simulink model "mainfile"  (R2016a)
settings: Solver=VariableStepAuto  StartTime=0.0  StopTime=3  RelTol=1e-3
undefined symbols (not defined in the file): Acid, Lead
libraries: powerlib x39, powerlib_meascontrol x6, simulink x3, electricdrivelib x1
settings Model: Creator=rinkesh.pee14  LastModifiedBy=rinkesh.pee14

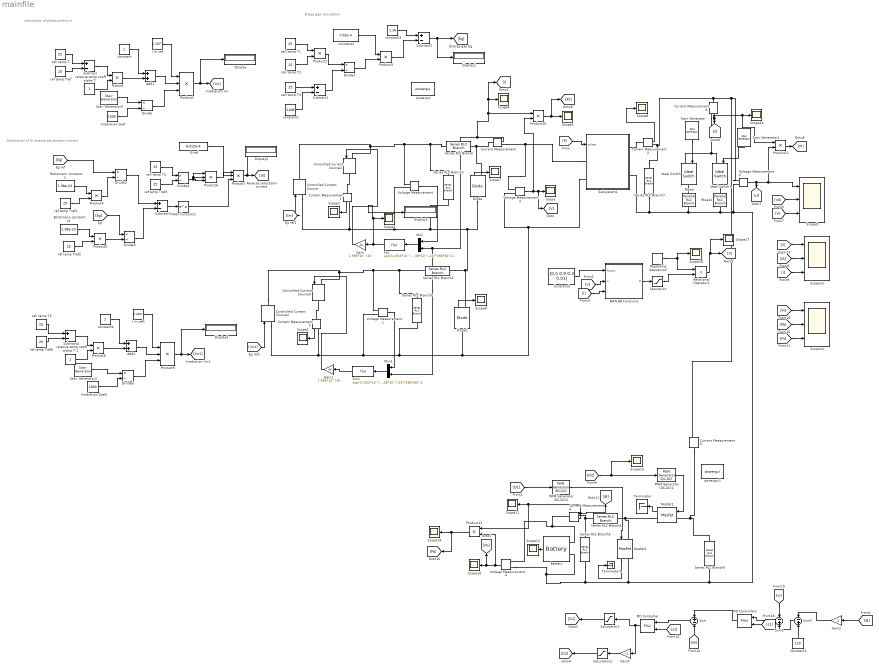
== system mainfile ==
  note: calculation of photocurrent Irr
  note: Enegy gap calculation
  note: Calculation of I0 reverse satuaration current
  Add1 : Sum
  Add2 : Sum
  Battery : electricdrivelib/Extra Sources/Battery  BatType=Lead-Acid  ShowTempParam=off  ThermalPreset=no  NomV=48  NomQ=50  SOC=50  Batt_Tr=30  PresetModel=on  MaxQ=52.0833  MinV=36  FullV=52.2632  Dis_rate=10  R=0.0096  Normal_OP=15.5139  expZone="[48.8684     0.166667]"  current=[1.5 3]  Units=Ampere-hour  Tci=20  NomT=20  T2=-30  MaxQ2=4.8  FullV2=7.1  Normal_OP2=5.655  expZone2="[6.58           1]"  Rca=0.6  ti=2000  Dp=0
  Boltzmann constant k : Constant  Value=1.38e-23
  Boltzmann constant k1 : Constant  Value=1.38e-23
  Constant1 : Constant  Value=120
  Constant3 : Constant  Value=[0.5 0.9 0.3 0.01]
  Controlled Current Source{,1..3} (4 alike) : powerlib/Electrical Sources/Controlled Current Source  Initialize=on  Source_Type=AC  Amplitude=0  Phase=0  Frequency=0  Measurements=None
  Current Measurement{,1..6} (7 alike) : powerlib/Measurements/Current Measurement  PhasorSimulation=off  OutputType=Complex  PSBequivalent=0
  Diode : powerlib/Power Electronics/Diode  Ron=0.001  Lon=0  Vf=0.8  IC=0  UseSnubber=off  Rs=500  Cs=250e-9  Measurements=on
  Diode1 : powerlib/Power Electronics/Diode  Ron=0.001  Lon=0  Vf=0.8  IC=0  UseSnubber=off  Rs=500  Cs=250e-9  Measurements=on
  Display{,1..3,5} (5 alike) : Display
  Divide{,1..5} (6 alike) : Product  Inputs=*/
  Fcn : Fcn  Expr=exp((1.602*10^(-19)*(u(1)+u(2)*0.01526*36))/(1.128*1.38*10^(-23)*298*36))-1
  Fcn1 : Fcn  Expr=exp((1.602*10^(-19)*(u(1)+u(2)*0.01526*36))/(1.128*1.38*10^(-23)*298*36))-1
  Gain : Gain  Gain=1.996*10^(-8)
  Gain1 : Gain  Gain=1.996*10^(-8)
  Gain2 : Gain  Gain=.1
  Gain3 : Gain  Gain=-1
  I irr,ref : Constant  Value=2.4207
  I irr,ref1 : Constant  Value=2.4207
  I0,ref : Constant  Value=6.012e-9
  Ideal Switch : powerlib/Power Electronics/Ideal Switch  Ron=0.001  Lon=0  IC=0  Rs=1e5  Cs=inf  Measurements=off
  Ideal Switch1 : powerlib/Power Electronics/Ideal Switch  Ron=0.001  Lon=0  IC=0  Rs=1e5  Cs=inf  Measurements=off
  Irradiation Gref : Constant  Value=1000
  Irradiation Gref1 : Constant  Value=1000
  MATLAB Function1 : MATLAB Function  TreatAsAtomicUnit=on
  Math Function1 : Math  SaturateOnIntegerOverflow=on
  Mosfet1 : powerlib/Power Electronics/Mosfet  Ron=0.1  Lon=0  Rd=0.01  Vfd=0  IC=0  Rs=1e5  Cs=inf  Measurements=on
  Mosfet2 : powerlib/Power Electronics/Mosfet  Ron=0.1  Lon=0  Rd=0.01  Vfd=0  IC=0  Rs=1e5  Cs=inf  Measurements=on
  Mux : Mux  Inputs=2
  Mux1 : Mux  Inputs=2
  PID Controller : simulink/Continuous/PID Controller  Controller=PI  TimeDomain=Continuous-time  SampleTime=-1  IntegratorMethod=Forward Euler  FilterMethod=Forward Euler  Form=Parallel  UseFilter=on  ControllerParametersSource=internal  P=.05  I=1  D=0.01  N=100  InitialConditionSource=internal  InitialConditionForIntegrator=0  InitialConditionForFilter=0  ExternalReset=either  ZeroCross=off  LimitOutput=off  UpperSaturationLimit=inf  LowerSaturationLimit=-inf  LinearizeAsGain=on  AntiWindupMode=none  Kb=1  TrackingMode=off  Kt=1  PParamMin=[]  PParamMax=[]  IParamMin=[]  IParamMax=[]  DParamMin=[]  DParamMax=[]  NParamMin=[]  NParamMax=[]  KbParamMin=[]  KbParamMax=[]  KtParamMin=[]  KtParamMax=[]  POutMin=[]  POutMax=[]  IOutMin=[]  IOutMax=[]  DOutMin=[]  DOutMax=[]  NOutMin=[]  NOutMax=[]  KbOutMin=[]  KbOutMax=[]  KtOutMin=[]  KtOutMax=[]  IntegratorOutMin=[]  IntegratorOutMax=[]  FilterOutMin=[]  FilterOutMax=[]  SumOutMin=[]  SumOutMax=[]  SumI1OutMin=[]  SumI1OutMax=[]  SumI2OutMin=[]  SumI2OutMax=[]  SumI3OutMin=[]  SumI3OutMax=[]  SumDOutMin=[]  SumDOutMax=[]  SaturationOutMin=[]  SaturationOutMax=[]  IntegratorContinuousStateAttributes=''  IntegratorStateMustResolveToSignalObject=off  IntegratorRTWStateStorageClass=Auto  FilterContinuousStateAttributes=''  FilterStateMustResolveToSignalObject=off  FilterRTWStateStorageClass=Auto  DifferentiatorICPrevScaledInput=0  DifferentiatorOutMin=[]  DifferentiatorOutMax=[]
  PID Controller1 : simulink/Continuous/PID Controller  Controller=PI  TimeDomain=Continuous-time  SampleTime=-1  IntegratorMethod=Forward Euler  FilterMethod=Forward Euler  Form=Ideal  UseFilter=on  ControllerParametersSource=internal  P=3  I=5  D=0.01  N=100  InitialConditionSource=internal  InitialConditionForIntegrator=0  InitialConditionForFilter=0  ExternalReset=either  ZeroCross=off  LimitOutput=off  UpperSaturationLimit=inf  LowerSaturationLimit=-inf  LinearizeAsGain=on  AntiWindupMode=none  Kb=1  TrackingMode=off  Kt=1  PParamMin=[]  PParamMax=[]  IParamMin=[]  IParamMax=[]  DParamMin=[]  DParamMax=[]  NParamMin=[]  NParamMax=[]  KbParamMin=[]  KbParamMax=[]  KtParamMin=[]  KtParamMax=[]  POutMin=[]  POutMax=[]  IOutMin=[]  IOutMax=[]  DOutMin=[]  DOutMax=[]  NOutMin=[]  NOutMax=[]  KbOutMin=[]  KbOutMax=[]  KtOutMin=[]  KtOutMax=[]  IntegratorOutMin=[]  IntegratorOutMax=[]  FilterOutMin=[]  FilterOutMax=[]  SumOutMin=[]  SumOutMax=[]  SumI1OutMin=[]  SumI1OutMax=[]  SumI2OutMin=[]  SumI2OutMax=[]  SumI3OutMin=[]  SumI3OutMax=[]  SumDOutMin=[]  SumDOutMax=[]  SaturationOutMin=[]  SaturationOutMax=[]  IntegratorContinuousStateAttributes=''  IntegratorStateMustResolveToSignalObject=off  IntegratorRTWStateStorageClass=Auto  FilterContinuousStateAttributes=''  FilterStateMustResolveToSignalObject=off  FilterRTWStateStorageClass=Auto  DifferentiatorICPrevScaledInput=0  DifferentiatorOutMin=[]  DifferentiatorOutMax=[]
  PWM Generator (DC-DC)1 : powerlib_meascontrol/Pulse & Signal Generators/PWM Generator (DC-DC)  Fsw=20000  Ts=0
  PWM Generator (DC-DC)2 : powerlib_meascontrol/Pulse & Signal Generators/PWM Generator (DC-DC)  Fsw=20000  Ts=0
  Product{,2..5,8,10..12} (9 alike) : Product  RndMeth=Zero
  Product{1,6..7,9} (4 alike) : Product  Inputs=3  RndMeth=Zero
  Relational Operator1 : RelationalOperator  Operator=<  OutDataTypeStr=boolean
  Repeating Sequence2 : simulink/Sources/Repeating Sequence  rep_seq_t=[0 0.0001]  rep_seq_y=[0 1]
  Rload : powerlib/Elements/Parallel RLC Branch  LConnTagsString=a  RConnTagsString=__new0  BranchType=R  Resistance=100  Inductance=1e-3  SetiL0=off  InitialCurrent=0  Capacitance=1e-6  Setx0=off  InitialVoltage=0  Measurements=None
  Rload1 : powerlib/Elements/Parallel RLC Branch  LConnTagsString=a  RConnTagsString=__new0  BranchType=R  Resistance=500  Inductance=1e-3  SetiL0=off  InitialCurrent=0  Capacitance=1e-6  Setx0=off  InitialVoltage=0  Measurements=None
  Saturation : Saturate  UpperLimit=1  LowerLimit=0
  Saturation1 : Saturate  UpperLimit=.9  LowerLimit=0
  Saturation2 : Saturate  UpperLimit=.9  LowerLimit=0
  Scope{,1..8,10..14,17..19} (17 alike) : Scope
  Scope15 : Scope  NumInputPorts=3
  Scope16 : Scope  NumInputPorts=3
  Scope9 : Scope  NumInputPorts=3
  Series RLC Branch : powerlib/Elements/Series RLC Branch  LConnTagsString=__new0  RConnTagsString=__new0  BranchType=R  Resistance=0.01526*36  Inductance=1e-3  SetiL0=off  InitialCurrent=0  Capacitance=1e-6  Setx0=off  InitialVoltage=0  Measurements=None
  Series RLC Branch1 : powerlib/Elements/Series RLC Branch  LConnTagsString=__new0  RConnTagsString=__new0  BranchType=R  Resistance=6.4616*36  Inductance=1e-3  SetiL0=off  InitialCurrent=0  Capacitance=1e-6  Setx0=off  InitialVoltage=0  Measurements=None
  Series RLC Branch2 : powerlib/Elements/Series RLC Branch  LConnTagsString=__new0  RConnTagsString=__new0  BranchType=R  Resistance=0.01526*36  Inductance=1e-3  SetiL0=off  InitialCurrent=0  Capacitance=1e-6  Setx0=off  InitialVoltage=0  Measurements=None
  Series RLC Branch3 : powerlib/Elements/Series RLC Branch  LConnTagsString=__new0  RConnTagsString=__new0  BranchType=R  Resistance=6.4616*36  Inductance=1e-3  SetiL0=off  InitialCurrent=0  Capacitance=1e-6  Setx0=off  InitialVoltage=0  Measurements=None
  Series RLC Branch4 : powerlib/Elements/Series RLC Branch  LConnTagsString=__new0  RConnTagsString=__new0  BranchType=L  Resistance=1  Inductance=1.5e-3  SetiL0=off  InitialCurrent=0  Capacitance=1e-6  Setx0=off  InitialVoltage=0  Measurements=None
  Series RLC Branch5 : powerlib/Elements/Series RLC Branch  LConnTagsString=__new0  RConnTagsString=__new0  BranchType=C  Resistance=0.1  Inductance=1e-3  SetiL0=off  InitialCurrent=0  Capacitance=1000e-4  Setx0=off  InitialVoltage=0  Measurements=None
  Series RLC Branch6 : powerlib/Elements/Series RLC Branch  LConnTagsString=__new0  RConnTagsString=__new0  BranchType=C  Resistance=0.001  Inductance=1e-3  SetiL0=off  InitialCurrent=0  Capacitance=3000e-6  Setx0=off  InitialVoltage=0  Measurements=None
  Series RLC Branch7 : powerlib/Elements/Series RLC Branch  LConnTagsString=__new0  RConnTagsString=__new0  BranchType=C  Resistance=0.001  Inductance=1e-3  SetiL0=off  InitialCurrent=0  Capacitance=2000e-6  Setx0=off  InitialVoltage=0  Measurements=None
  Stair Generator : powerlib_meascontrol/Pulse & Signal Generators/Stair Generator  t=[0, 2.5]  e=[1,0]  Ts=0
  Stair Generator1 : powerlib_meascontrol/Pulse & Signal Generators/Stair Generator  t=[0]  e=[1]  Ts=0
  Stair Generator2 : powerlib_meascontrol/Pulse & Signal Generators/Stair Generator  t=[0, 1.5]  e=[1000,00]  Ts=0
  Stair Generator3 : powerlib_meascontrol/Pulse & Signal Generators/Stair Generator  t=[0, 1.5]  e=[1000,00]  Ts=0
  Subsystem1 : Subsystem
  Subtract{,1..4} (5 alike) : Sum  Inputs=+-
  Sum : Sum  Inputs=+-
  Sum1 : Sum  Inputs=-+
  Sum2 : Sum  Inputs=-+
  Terminator : Terminator
  Terminator1 : Terminator
  Voltage Measurement{,1..4} (5 alike) : powerlib/Measurements/Voltage Measurement  PhasorSimulation=off  OutputType=Complex  PSBequivalent=0
  cell temp T{,1..5} (6 alike) : Constant  Value=25
  constant : Constant
  constant1 : Constant  Value=1108
  constant2 : Constant  Value=7.02e-4  VectorParams1D=off
  constant3 : Constant  Value=1.16
  constant4 : Constant
  powergui : powerlib/powergui  Priority=1  SimulationMode=Discrete  SolverType=Tustin/Backward Euler (TBE)  SampleTime=1e-6  frequency=60  SPID=off  DisableSnubberDevices=off  DisableRonSwitches=off  DisableVfSwitches=off  SwTol=0  DisplayEquations=off  Interpol=off  ExternalGateDelay=off  methode=off  Ts=0  FunctionMessages=off  echomessages=off  HookPort=off  EnableUseOfTLC=off  x0status=blocks  frequencyindice=0  Pbase=100e6  ErrMax=1e-4  Iterations=50  UnitsV=kV  UnitsW=MW  buscounter=0  RestoreLinks=warning  ResistiveCurrentMeasurement=off  Frange=[0:2:500]  Ylog=off  Xlog=on  ShowGrid=off  save=off  variable=ZData  structure=0  ZoomFFT=off  StartTime=0.0  cycles=1  DisplayStyle=1  fundamental=60  FreqAxis=off  MaxFrequency=1000  frequencyindicesteady=1  RmsSteady=1  display=off
  powergui1 : powerlib/powergui  Priority=1  SimulationMode=Continuous  SolverType=Tustin  SampleTime=50e-6  frequency=60  SPID=off  DisableSnubberDevices=off  DisableRonSwitches=off  DisableVfSwitches=off  SwTol=0  DisplayEquations=off  Interpol=off  ExternalGateDelay=off  methode=off  Ts=0  FunctionMessages=off  echomessages=off  HookPort=off  EnableUseOfTLC=off  x0status=blocks  frequencyindice=0  Pbase=100e6  ErrMax=1e-4  Iterations=50  UnitsV=kV  UnitsW=MW  buscounter=0  RestoreLinks=warning  ResistiveCurrentMeasurement=off  Frange=[0:2:500]  Ylog=off  Xlog=on  ShowGrid=off  save=off  variable=ZData  structure=0  ZoomFFT=off  StartTime=0.0  cycles=1  DisplayStyle=1  fundamental=60  FreqAxis=off  MaxFrequency=1000  frequencyindicesteady=1  RmsSteady=1  display=off
  ref temp Tref{,1..4} (5 alike) : Constant  Value=25
  "relative temp coeff alpha T' " : Constant
  relative temp coeff alpha T' 1 : Constant
  wires:
  cell temp T/1 -> Subtract/1
  ref temp Tref/1 -> Subtract/2
  Subtract/1 -> Product/1
  "relative temp coeff alpha T' "/1 -> Product/2
  Product/1 -> Add1/2
  constant/1 -> Add1/1
  Stair Generator3/1 -> Divide/1
  Irradiation Gref/1 -> Divide/2
  Add1/1 -> Product1/2
  Divide/1 -> Product1/3
  I irr,ref/1 -> Product1/1
  cell temp T1/1 -> Product2/1
  cell temp T2/1 -> Product2/2
  cell temp T3/1 -> Subtract1/1
  constant1/1 -> Subtract1/2
  Product2/1 -> Divide1/1
  Subtract1/1 -> Divide1/2
  constant2/1 -> Product3/1
  Divide1/1 -> Product3/2
  constant3/1 -> Subtract2/1
  Product3/1 -> Subtract2/2
  Product1/1 -> [Iirr], Display/1
  Subtract2/1 -> [Eg], Display1/1
  Boltzmann constant k/1 -> Product4/1
  ref temp Tref1/1 -> Product4/2
  [Eg] -> Divide2/1
  Product4/1 -> Divide2/2
  Boltzmann constant k1/1 -> Product5/1
  ref temp Tref2/1 -> Product5/2
  Product5/1 -> Divide3/2
  [Eg] -> Divide3/1
  Divide2/1 -> Subtract3/1
  Divide3/1 -> Subtract3/2
  Subtract3/1 -> Math Function1/1
  cell temp T4/1 -> Divide4/1
  ref temp Tref3/1 -> Divide4/2
  Divide4/1 -> Product6/3, Product6/2, Product6/1
  Math Function1/1 -> Product7/3
  Product6/1 -> Product7/2
  I0,ref/1 -> Product7/1
  Product7/1 -> [I0], Display2/1
  [Iirr] -> Controlled Current Source/1
  Fcn/1 -> Gain/1, Scope3/1, Display5/1
  Gain/1 -> Controlled Current Source1/1
  Mux/1 -> Fcn/1
  Current Measurement1/1 -> Scope2/1
  cell temp T5/1 -> Subtract4/1
  ref temp Tref4/1 -> Subtract4/2
  Subtract4/1 -> Product8/1
  relative temp coeff alpha T' 1/1 -> Product8/2
  Product8/1 -> Add2/2
  constant4/1 -> Add2/1
  Stair Generator2/1 -> Divide5/1
  Irradiation Gref1/1 -> Divide5/2
  Add2/1 -> Product9/2
  Divide5/1 -> Product9/3
  I irr,ref1/1 -> Product9/1
  Product9/1 -> [Iirr1], Display3/1
  [Iirr1] -> Controlled Current Source2/1
  Fcn1/1 -> Gain1/1
  Gain1/1 -> Controlled Current Source3/1
  Mux1/1 -> Fcn1/1
  Current Measurement3/1 -> Scope1/1
  Voltage Measurement1/1 -> Mux1/1
  Voltage Measurement/1 -> Mux/1
  Current Measurement/1 -> Mux/2, Mux1/2, Scope4/1, [I], Product10/1
  Voltage Measurement3/1 -> Product10/2, [V], Scope/1
  Product10/1 -> [Ps], Scope5/1
  Diode1/1 -> Scope6/1
  Diode/1 -> Scope7/1
  Current Measurement2/1 -> Scope8/1
  [P] -> Subsystem1/1("pulses ")
  Voltage Measurement2/1 -> Product11/2, Scope9/1, [vl]
  Constant3/1 -> MATLAB Function1/1(Param)
  Repeating Sequence2/1 -> Scope18/1, Relational Operator1/1
  MATLAB Function1/1(D) -> Saturation/1
  [V] -> MATLAB Function1/2(V)
  [I] -> MATLAB Function1/3(I)
  Relational Operator1/1 -> Scope17/1, [P]
  Saturation/1 -> Relational Operator1/2
  [D1] -> PWM Generator (DC-DC)2/1
  PWM Generator (DC-DC)2/1 -> Mosfet2/1
  Mosfet2/1 -> Terminator1/1
  PWM Generator (DC-DC)1/1 -> Mosfet1/1
  Mosfet1/1 -> Terminator/1
  Battery/1 -> Scope12/1
  [D2] -> Scope13/1, PWM Generator (DC-DC)1/1
  PID Controller/1 -> Gain3/1, Saturation1/1
  Saturation1/1 -> [D1]
  Sum1/1 -> PID Controller1/1
  Sum2/1 -> Sum1/2
  PID Controller1/1 -> Sum/1
  Sum/1 -> PID Controller/1
  Gain2/1 -> Sum2/1
  Constant1/1 -> Sum2/2
  Stair Generator1/1 -> Ideal Switch1/1
  [iB] -> Gain2/1
  [iB] -> Sum/2
  [vl] -> Sum1/1
  [s1] -> PID Controller/2
  [s1] -> PID Controller1/2
  Current Measurement6/1 -> Product11/1, Scope14/1, [il]
  Stair Generator/1 -> Ideal Switch/1
  Saturation2/1 -> [D2]
  Gain3/1 -> Saturation2/1
  Current Measurement4/1 -> [iB], Product12/1, Scope11/1
  [Vb] -> Scope9/2
  [V] -> Scope9/3
  [iB] -> Scope15/2
  [I] -> Scope15/3
  [Pb] -> Scope16/2
  [Ps] -> Scope16/3
  [il] -> Scope15/1
  [Pl] -> Scope16/1
  Product11/1 -> [Pl]
  Voltage Measurement4/1 -> Product12/2, [Vb], Scope10/1
  Product12/1 -> [Pb], Scope19/1
  connections:
  Series RLC Branch1/LConn1 -- Series RLC Branch/LConn1 -- Controlled Current Source/RConn1 -- Controlled Current Source1/LConn1 -- Voltage Measurement/LConn1
  Series RLC Branch/RConn1 -- Current Measurement/LConn1 -- Diode/RConn1
  Controlled Current Source2/RConn1 -- Controlled Current Source3/LConn1 -- Voltage Measurement1/LConn1 -- Series RLC Branch2/LConn1 -- Series RLC Branch3/LConn1
  Voltage Measurement1/LConn2 -- Controlled Current Source2/LConn1 -- Current Measurement3/RConn1 -- Voltage Measurement3/LConn2 -- Subsystem1/LConn2 -- Diode1/LConn1 -- Series RLC Branch3/RConn1
  Diode/LConn1 -- Series RLC Branch1/RConn1 -- Voltage Measurement/LConn2 -- Controlled Current Source/LConn1 -- Current Measurement1/RConn1 -- Series RLC Branch2/RConn1 -- Diode1/RConn1
  Subsystem1/LConn1 -- Current Measurement/RConn1 -- Voltage Measurement3/LConn1
  Subsystem1/RConn2 -- Series RLC Branch7/LConn1 -- Rload/RConn1 -- Rload1/RConn1 -- Voltage Measurement2/LConn2 -- Series RLC Branch6/LConn1 -- Mosfet2/RConn1 -- Voltage Measurement4/LConn2 -- Battery/LConn2 -- Series RLC Branch5/LConn1
  Mosfet1/RConn1 -- Series RLC Branch4/RConn1 -- Mosfet2/LConn1
  Series RLC Branch5/RConn1 -- Current Measurement4/RConn1 -- Series RLC Branch4/LConn1
  Battery/LConn1 -- Current Measurement4/LConn1 -- Voltage Measurement4/LConn1
  Mosfet1/LConn1 -- Series RLC Branch6/RConn1 -- Current Measurement5/LConn1
  Series RLC Branch7/RConn1 -- Current Measurement2/RConn1 -- Current Measurement6/LConn1 -- Current Measurement5/RConn1 -- Voltage Measurement2/LConn1
  Ideal Switch/LConn1 -- Current Measurement6/RConn1 -- Ideal Switch1/LConn1
  Current Measurement1/LConn1 -- Controlled Current Source1/RConn1
  Current Measurement3/LConn1 -- Controlled Current Source3/RConn1
  Current Measurement2/LConn1 -- Subsystem1/RConn1
  Ideal Switch/RConn1 -- Rload/LConn1
  Ideal Switch1/RConn1 -- Rload1/LConn1

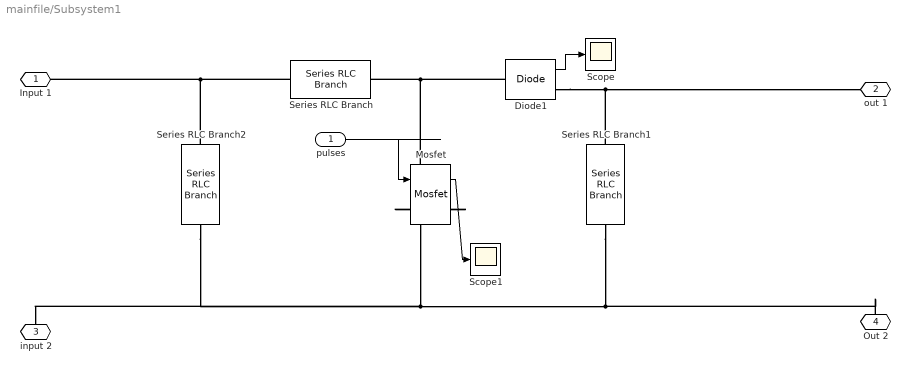
== system mainfile/Subsystem1 ==
  "pulses " : Inport
  Diode1 : powerlib/Power Electronics/Diode  Ron=0.001  Lon=0  Vf=0.8  IC=0  UseSnubber=off  Rs=500  Cs=250e-9  Measurements=on
  Mosfet : powerlib/Power Electronics/Mosfet  Ron=0.1  Lon=0  Rd=0.01  Vfd=0  IC=0  Rs=1e5  Cs=inf  Measurements=on
  Scope : Scope
  Scope1 : Scope
  Series RLC Branch : powerlib/Elements/Series RLC Branch  LConnTagsString=__new0  RConnTagsString=__new0  BranchType=L  Resistance=1  Inductance=100e-3  SetiL0=off  InitialCurrent=0  Capacitance=1e-6  Setx0=off  InitialVoltage=0  Measurements=None
  Series RLC Branch1 : powerlib/Elements/Series RLC Branch  LConnTagsString=__new0  RConnTagsString=__new0  BranchType=C  Resistance=1  Inductance=50e-3  SetiL0=on  InitialCurrent=0  Capacitance=200e-6  Setx0=off  InitialVoltage=0  Measurements=None
  Series RLC Branch2 : powerlib/Elements/Series RLC Branch  LConnTagsString=__new0  RConnTagsString=__new0  BranchType=C  Resistance=1  Inductance=50e-3  SetiL0=on  InitialCurrent=0  Capacitance=200e-6  Setx0=off  InitialVoltage=0  Measurements=None
  Input 1 : PMIOPort  Port=1  Side=Left
  out 1 : PMIOPort  Port=2  Side=Right
  input 2 : PMIOPort  Port=3  Side=Left
  Out 2 : PMIOPort  Port=4  Side=Right
  wires:
  Diode1/1 -> Scope/1
  Mosfet/1 -> Scope1/1
  "pulses "/1 -> Mosfet/1
  connections:
  Series RLC Branch/LConn1 -- Series RLC Branch2/LConn1 -- Input 1/RConn1
  Diode1/RConn1 -- out 1/RConn1 -- Series RLC Branch1/LConn1
  Diode1/LConn1 -- Mosfet/LConn1 -- Series RLC Branch/RConn1
  Series RLC Branch1/RConn1 -- Out 2/RConn1 -- input 2/RConn1 -- Series RLC Branch2/RConn1 -- Mosfet/RConn1

== matlab function mainfile/MATLAB Function1 ==
  data: Param input; D output; V input; I input
function D  = PandO(Param, V, I)

% MPPT controller based on the Perturb & Observe algorithm.

% D output = Duty cycle of the boost converter (value between 0 and 1)
%
% Enabled input = 1 to enable the MPPT controller
% V input = PV array terminal voltage (V)
% I input = PV array current (A)
%
% Param input:
Dinit = Param(1);  %Initial value for D output
Dmax = Param(2);   %Maximum value for D
Dmin = Param(3);   %Minimum value for D
deltaD = Param(4); %Increment value used to increase/decrease the duty cycle D
% ( increasing D = decreasing Vref )
%  

persistent Vold Pold Dold;

dataType = 'double';

if isempty(Vold)
    Vold=0;
    Pold=0;
    Dold=Dinit;
end
P= V*I;
dV= V - Vold;
dP= P - Pold;

if dP ~= 0
    if dP < 0
        if dV < 0
            D = Dold - deltaD;
        else
            D = Dold + deltaD;
        end
    else
        if dV < 0
            D = Dold + deltaD;
        else
            D = Dold - deltaD;
        end    
    end
else D=Dold;
end

if D >= Dmax | D<= Dmin
    D=Dold;
end

Dold=D;
Vold=V;
Pold=P;
